simulink library "limblab"  (Simulink 6.6)
libraries: xpclib x4, simulink x4, limblab x1
settings Model: Creator=limblab  LastModifiedBy=system administrator

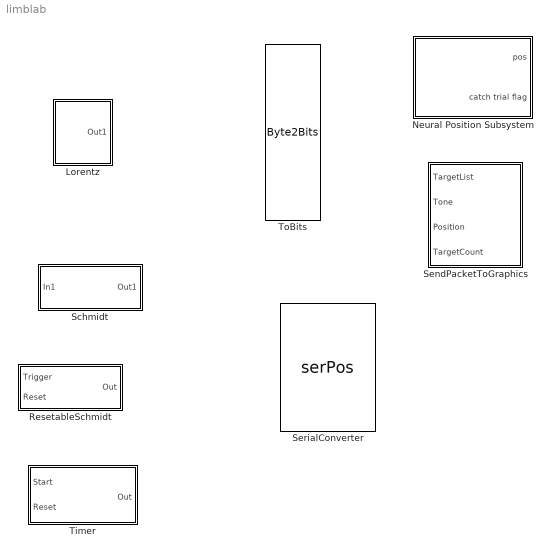
== system limblab ==
  Lorentz : Subsystem  mask(Lorentz attractor){y0=.1}
      mask prompts: y0 "Initial Condition"
      mask help: Creats chaotic oscelations using a lorentz attractor algorithm.
      mask Help:
      | Creats chaotic oscelations using a lorentz attractor algorithm.
      | 
      | This particular oscilator has the parameters:
      | rho = 28
      | beta = 8/3
      | sigma = 10
      | 
      | The initial condition y0 can be specified as a parameter.
      | 
      | Other initial conditions (x0 and z0) are 0.1.
      mask Display: port_label('output', 1, 'Out')
  Neural Position Subsystem : Subsystem  SystemSampleTime=0.01
      mask Type: Neural Position Subsystem
      mask Description: Uses a UDP receive block to receive and parse the sent neural position from the real time system.
      mask Display:
      | port_label('output',1,'pos')
      | port_label('output',2,'catch trial flag')
  ResetableSchmidt : Subsystem  mask{Time=3}
  Schmidt : Subsystem  mask(Schmidt Trigger){Time=.3}
      mask help: Creates an output pulse of the specified time in seconds when trig goes high
      mask Help: Creates an output pulse of the specified time in seconds when trig goes high
      mask Display:
      | port_label('output',1,'out')
      | port_label('input',1,'trig')
      | fprintf('t = %.2f',Time)
  SendPacketToGraphics : Subsystem
  SerialConverter : S-Function  FunctionName=serPos
      mask Display:
      | port_label('output', 1, 'Byte Out')
      | port_label('input', 1, 'index')
      | port_label('input', 2, 'sh')
      | port_label('input', 3, 'el')
  Timer : Subsystem  mask{Time=.1}
      mask prompts: Time "Timeout"
      mask Display:
      | port_label('output',1,'out')
      | port_label('input',1,'start')
      | port_label('input',2,'reset')
      | fprintf('t = %.2f',Time)
  ToBits : S-Function  FunctionName=Byte2Bits
      mask Display:
      | port_label('input', 1, 'u')
      | port_label('output', 1, 'y0')
      | port_label('output', 2, 'y1')
      | port_label('output', 3, 'y2')
      | port_label('output', 4, 'y3')
      | port_label('output', 5, 'y4')
      | port_label('output', 6, 'y5')
      | port_label('output', 7, 'y6')
      | port_label('output', 8, 'y7')

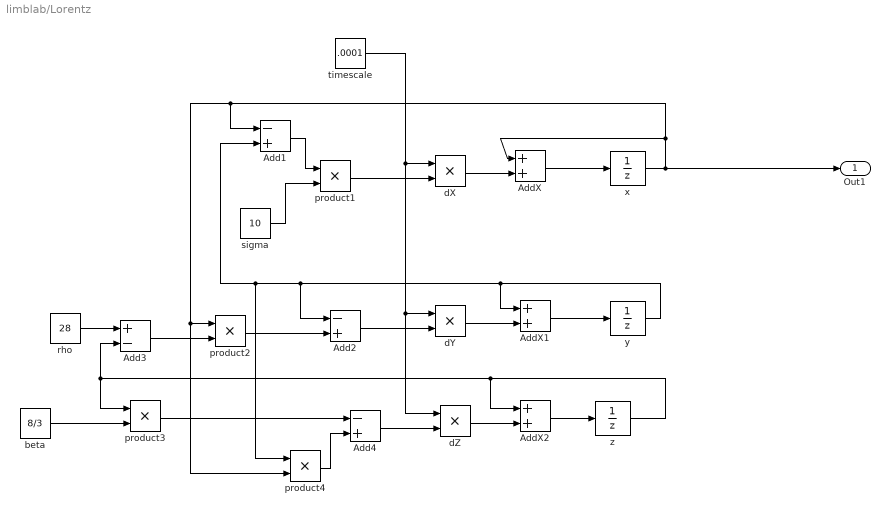
== system limblab/Lorentz ==
  Add1 : Sum  Inputs=-+  OutScaling=2^-10
  Add2 : Sum  Inputs=-+  OutScaling=2^-10
  Add3 : Sum  Inputs=+-  OutScaling=2^-10
  Add4 : Sum  Inputs=-+  OutScaling=2^-10
  AddX : Sum  OutScaling=2^-10
  AddX1 : Sum  OutScaling=2^-10
  AddX2 : Sum  OutScaling=2^-10
  beta : Constant  Value=8/3
  dX : Product  RndMeth=Zero
  dY : Product  RndMeth=Zero
  dZ : Product  RndMeth=Zero
  product{1..4} (4 alike) : Product  RndMeth=Zero
  rho : Constant  Value=28
  sigma : Constant  Value=10
  timescale : Constant  Value=.0001
  x : UnitDelay  X0=.1  SampleTime=.001
  y : UnitDelay  X0=y0  SampleTime=.001
  z : UnitDelay  X0=.1  SampleTime=.001
  Out1 : Outport
  wires:
  AddX/1 -> x/1
  AddX1/1 -> y/1
  AddX2/1 -> z/1
  y/1 -> AddX1/1, Add2/1, Add1/2, product4/1
  z/1 -> AddX2/1, Add3/2, product3/1
  x/1 -> Out1/1, AddX/1, Add1/1, product2/1, product4/2
  dX/1 -> AddX/2
  dY/1 -> AddX1/2
  dZ/1 -> AddX2/2
  timescale/1 -> dX/1, dY/1, dZ/1
  sigma/1 -> product1/2
  product1/1 -> dX/2
  Add1/1 -> product1/1
  Add2/1 -> dY/2
  product2/1 -> Add2/2
  Add3/1 -> product2/2
  rho/1 -> Add3/1
  beta/1 -> product3/2
  product3/1 -> Add4/1
  product4/1 -> Add4/2
  Add4/1 -> dZ/2

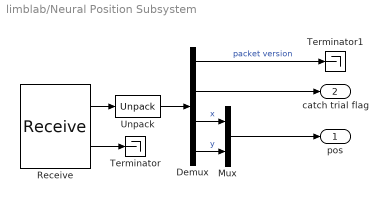
== system limblab/Neural Position Subsystem ==
  Demux : Demux
  Mux : Mux  Inputs=2
  Receive : xpclib/UDP/Receive  ipAddress=0.0.0.0  ipPort=24999  width=16  sampletime=0.001
  Terminator : Terminator
  Terminator1 : Terminator
  Unpack : xpclib/UDP/Unpack  dimensions={[1,4]}  datatypes={'single'}  byteAlign=1
  pos : Outport
  catch trial flag : Outport  Port=2
  wires:
  Demux/2 -> catch trial flag/1
  Mux/1 -> pos/1
  Demux/4 -> Mux/2  "y"
  Demux/3 -> Mux/1  "x"
  Demux/1 -> Terminator1/1  "packet version"
  Unpack/1 -> Demux/1
  Receive/2 -> Terminator/1
  Receive/1 -> Unpack/1

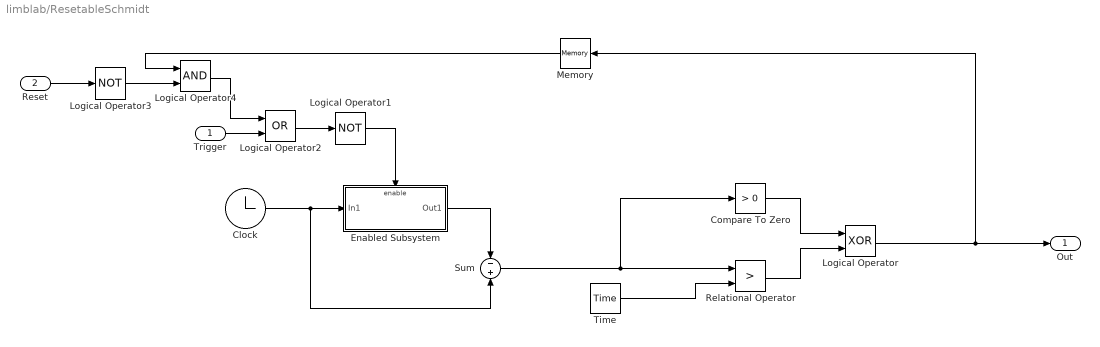
== system limblab/ResetableSchmidt ==
  Trigger : Inport
  Reset : Inport  Port=2
  Clock : Clock
  Compare To Zero : simulink/Logic and Bit Operations/Compare To Zero  SystemSampleTime=-1  relop=>  LogicOutDataTypeMode=uint8  ZeroCross=off
  Enabled Subsystem : Subsystem  TreatAsAtomicUnit=on
  Logical Operator : Logic  Operator=XOR  AllPortsSameDT=off  OutDataTypeMode=Boolean  SampleTime=.001
  Logical Operator1 : Logic  Operator=NOT  AllPortsSameDT=off  OutDataTypeMode=Boolean
  Logical Operator2 : Logic  Operator=OR  AllPortsSameDT=off  OutDataTypeMode=Boolean  SampleTime=.001
  Logical Operator3 : Logic  Operator=NOT  AllPortsSameDT=off  OutDataTypeMode=Boolean
  Logical Operator4 : Logic  AllPortsSameDT=off  OutDataTypeMode=Boolean  SampleTime=.001
  Memory : Memory  Orientation=left
  Relational Operator : RelationalOperator  Operator=>  LogicOutDataTypeMode=Boolean
  Sum : Sum  Inputs=-+
  Time : Constant  Value=Time
  Out : Outport
  wires:
  Logical Operator2/1 -> Logical Operator1/1
  Trigger/1 -> Logical Operator2/2
  Logical Operator/1 -> Memory/1, Out/1
  Logical Operator1/1 -> Enabled Subsystem/Enable
  Relational Operator/1 -> Logical Operator/2
  Compare To Zero/1 -> Logical Operator/1
  Time/1 -> Relational Operator/2
  Sum/1 -> Relational Operator/1, Compare To Zero/1
  Enabled Subsystem/1(Out1) -> Sum/1
  Clock/1 -> Sum/2, Enabled Subsystem/1(In1)
  Reset/1 -> Logical Operator3/1
  Logical Operator3/1 -> Logical Operator4/2
  Logical Operator4/1 -> Logical Operator2/1
  Memory/1 -> Logical Operator4/1

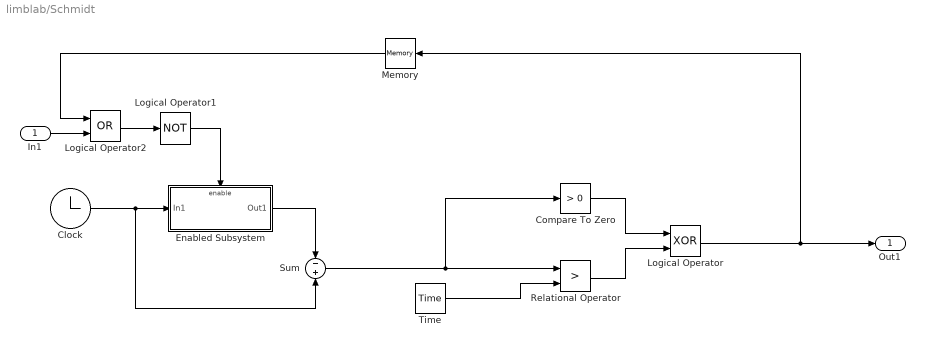
== system limblab/Schmidt ==
  In1 : Inport
  Clock : Clock
  Compare To Zero : simulink/Logic and Bit Operations/Compare To Zero  SystemSampleTime=-1  relop=>  LogicOutDataTypeMode=uint8  ZeroCross=off
  Enabled Subsystem : Subsystem  TreatAsAtomicUnit=on
  Logical Operator : Logic  Operator=XOR  AllPortsSameDT=off  OutDataTypeMode=Boolean  SampleTime=.001
  Logical Operator1 : Logic  Operator=NOT  AllPortsSameDT=off  OutDataTypeMode=Boolean
  Logical Operator2 : Logic  Operator=OR  AllPortsSameDT=off  OutDataTypeMode=Boolean  SampleTime=.001
  Memory : Memory  Orientation=left
  Relational Operator : RelationalOperator  Operator=>  LogicOutDataTypeMode=Boolean
  Sum : Sum  Inputs=-+
  Time : Constant  Value=Time
  Out1 : Outport
  wires:
  Clock/1 -> Enabled Subsystem/1(In1), Sum/2
  Enabled Subsystem/1(Out1) -> Sum/1
  Sum/1 -> Compare To Zero/1, Relational Operator/1
  Time/1 -> Relational Operator/2
  Compare To Zero/1 -> Logical Operator/1
  Relational Operator/1 -> Logical Operator/2
  Logical Operator1/1 -> Enabled Subsystem/Enable
  Logical Operator/1 -> Out1/1, Memory/1
  In1/1 -> Logical Operator2/2
  Logical Operator2/1 -> Logical Operator1/1
  Memory/1 -> Logical Operator2/1

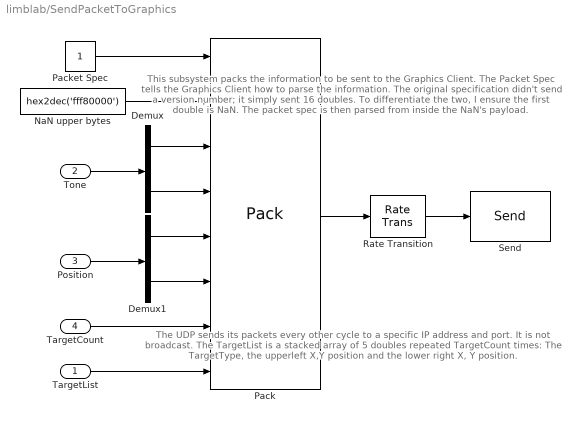
== system limblab/SendPacketToGraphics ==
  note: This subsystem packs the information
      | to be sent to the Graphics Client.  The
      | Packet Spec tells the Graphics Client
      | how to parse the information.  The
      | original specification didn't send a version
      | number; it simply sent 16 doubles.  To
      | differentiate the two, I ensure the first
      | double is NaN.  The packet spec is then
      | parsed from inside the NaN's payload.
  note: The UDP sends its packets every other cycle
      | to a specific IP address and port.  It is not
      | broadcast.
      |
      | The TargetList is a stacked array
      | of 5 doubles repeated TargetCount times:
      | The TargetType, the upperleft X,Y position
      | and the lower right X, Y position.
  TargetList : Inport
  Tone : Inport  Port=2  PortDimensions=[2]
  Position : Inport  Port=3  PortDimensions=[2]
  TargetCount : Inport  Port=4  PortDimensions=[1]
  Demux : Demux  Outputs=2
  Demux1 : Demux  Outputs=2
  NaN upper bytes : Constant  Value=hex2dec('fff80000')  OutDataTypeMode=uint32
  Pack : xpclib/UDP/Pack  datatypes={'uint32','uint32','double','double','double','double','double','double'}  byteAlign=1
  Packet Spec : Constant  OutDataTypeMode=uint32
  Rate Transition : RateTransition
  Send : xpclib/UDP/Send  ipAddress=192.168.0.2  ipPort=25000  localPort=-1  sampletime=.02
  wires:
  Rate Transition/1 -> Send/1
  Pack/1 -> Rate Transition/1
  Tone/1 -> Demux/1
  Position/1 -> Demux1/1
  TargetList/1 -> Pack/8
  TargetCount/1 -> Pack/7
  Demux1/2 -> Pack/6
  Demux1/1 -> Pack/5
  Demux/2 -> Pack/4
  Demux/1 -> Pack/3
  NaN upper bytes/1 -> Pack/2
  Packet Spec/1 -> Pack/1

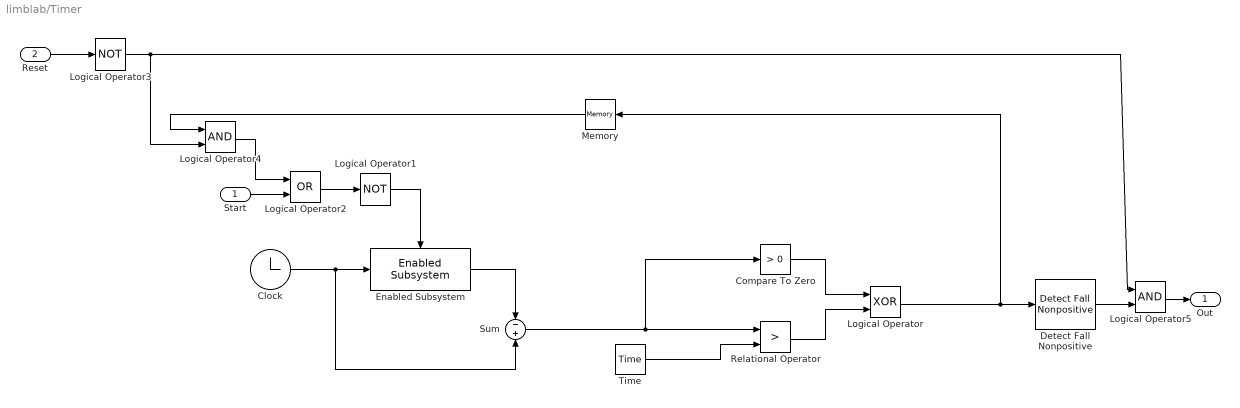
== system limblab/Timer ==
  Start : Inport
  Reset : Inport  Port=2
  Clock : Clock
  Compare To Zero : simulink/Logic and Bit Operations/Compare To Zero  SystemSampleTime=-1  relop=>  LogicOutDataTypeMode=uint8  ZeroCross=off
  Detect Fall Nonpositive : simulink/Logic and Bit Operations/Detect Fall Nonpositive  SystemSampleTime=-1  vinit=0
  Enabled Subsystem : limblab/ResetableSchmidt/Enabled Subsystem  SystemSampleTime=-1
  Logical Operator : Logic  Operator=XOR  AllPortsSameDT=off  OutDataTypeMode=Boolean  SampleTime=.001
  Logical Operator1 : Logic  Operator=NOT  AllPortsSameDT=off  OutDataTypeMode=Boolean
  Logical Operator2 : Logic  Operator=OR  AllPortsSameDT=off  OutDataTypeMode=Boolean  SampleTime=.001
  Logical Operator3 : Logic  Operator=NOT  AllPortsSameDT=off  OutDataTypeMode=Boolean
  Logical Operator4 : Logic  AllPortsSameDT=off  OutDataTypeMode=Boolean  SampleTime=.001
  Logical Operator5 : Logic  AllPortsSameDT=off  OutDataTypeMode=Boolean  SampleTime=.001
  Memory : Memory  Orientation=left
  Relational Operator : RelationalOperator  Operator=>  LogicOutDataTypeMode=Boolean
  Sum : Sum  Inputs=-+
  Time : Constant  Value=Time
  Out : Outport
  wires:
  Memory/1 -> Logical Operator4/1
  Logical Operator4/1 -> Logical Operator2/1
  Logical Operator3/1 -> Logical Operator5/1, Logical Operator4/2
  Reset/1 -> Logical Operator3/1
  Clock/1 -> Sum/2, Enabled Subsystem/1
  Enabled Subsystem/1 -> Sum/1
  Sum/1 -> Relational Operator/1, Compare To Zero/1
  Time/1 -> Relational Operator/2
  Compare To Zero/1 -> Logical Operator/1
  Relational Operator/1 -> Logical Operator/2
  Logical Operator1/1 -> Enabled Subsystem/Enable
  Logical Operator/1 -> Memory/1, Detect Fall Nonpositive/1
  Start/1 -> Logical Operator2/2
  Logical Operator2/1 -> Logical Operator1/1
  Detect Fall Nonpositive/1 -> Logical Operator5/2
  Logical Operator5/1 -> Out/1

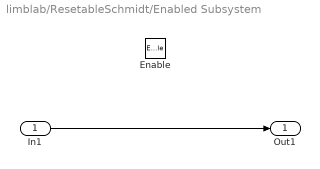
== system limblab/ResetableSchmidt/Enabled Subsystem ==
  In1 : Inport
  Enable : EnablePort
  Out1 : Outport
  wires:
  In1/1 -> Out1/1

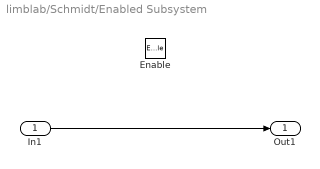
== system limblab/Schmidt/Enabled Subsystem ==
  In1 : Inport
  Enable : EnablePort
  Out1 : Outport
  wires:
  In1/1 -> Out1/1
